simulink model "Experiment_cs"  (Simulink 8.4)
settings: Solver=ode5  SolverMode=SingleTasking  StartTime=0.0  StopTime=inf  FixedStep=1/100  RelTol=1e-3
PreLoadFcn:
  | mbxruntime.callbacks.PreLoadFcn(bdroot);
PostLoadFcn:
  | mbxruntime.callbacks.PostLoadFcn(bdroot);
InitFcn:
  | mbxruntime.callbacks.InitFcn(bdroot);
StartFcn:
  | mbxruntime.callbacks.StartFcn(bdroot);
StopFcn:
  | mbxruntime.callbacks.StopFcn(bdroot);
undefined symbols (not defined in the file or in its folder): dfreq, gray, InitImageOutputDir, Rec, SDTV, strel
libraries: simulink x79, visiontextngfix x30, simulink_extras x23, PreScanSimulinkLibrary x20, visionconversions x6, visionsinks x4, PreScanUsefulBlocks x3, visionstatistics x2, visionmorphops x2, visionanalysis x2, simulink_need_slupdate x2
(part 8 of 11)

== system Experiment_cs/Audi_A8_1/ENABLED/Dynamics_Simple/Chassis/Bicycle_model_[XYZ]/X_Motion ==
  DriveTorque_[Nm] : Inport
  BrakePressure_[bar] : Inport  Port=2
  v0_[ms-1] : Inport  Port=3
  Air&RoadResistance : Subsystem
  BrakeSystem : Subsystem
  Configurable Subsystem : Subsystem  BlockChoice=Integrator  mask{ComputationMode=ComputationMode}
      mask prompts: ComputationMode "Computation mode:"
      mask init:
      | SetComputationMode(gcb,ComputationMode);
      settings: AttributesFormatString=%<BlockChoice>  OpenFcn=BringToFront(gcb);  MemberBlocks=Discrete-Time Integrator,Integrator
      settings: TemplateBlock=|
      | PreScanSimulinkLibrary/Configurable Subsystems/integral with reset and initial condition/Configurable
      | Subsystem
  Configurable Subsystem1 : Subsystem  BlockChoice=Torsional damping  mask{ComputationMode=ComputationMode}
      mask prompts: ComputationMode "Compuation mode:"
      mask init:
      | SetComputationMode(gcb,ComputationMode);
      settings: AttributesFormatString=%<BlockChoice>  OpenFcn=BringToFront(gcb);  MemberBlocks=Discrete Torsional damping,Torsional damping
      settings: TemplateBlock=|
      | PreScanSimulinkLibrary/Configurable Subsystems/TransferFunction
      | Torsional damping/Configurable
      | Subsystem
  Gain : Gain  Gain=1/p.Rw
  Inertia : Gain  Gain=1/p.m  SaturateOnIntegerOverflow=on  OutDataTypeStr=Inherit: Same as input  ParamDataTypeStr=Inherit: Same as input
  Max RPM and zero- velocity detection : Subsystem
  Sum : Sum  Inputs=+-  SaturateOnIntegerOverflow=on  InputSameDT=on  OutDataTypeStr=Inherit: Same as first input
  Sum2 : Sum  Inputs=+-  SaturateOnIntegerOverflow=on  InputSameDT=on  OutDataTypeStr=Inherit: Same as first input
  vx_[ms-1] : Outport
  ax_[ms-2] : Outport  Port=2
  wires:
  Sum/1 -> Sum2/1  "sumForce_[N]"
  Inertia/1 -> Max RPM and zero- velocity detection/1(ax)  "ax[ms-2]"
  Sum2/1 -> Inertia/1
  Air&RoadResistance/1(Resistance_Force) -> Sum/2
  Configurable Subsystem/1(Out1) -> vx_[ms-1]/1, Air&RoadResistance/1(vx_[ms-1]), BrakeSystem/1(vx_[ms-1]), Max RPM and zero- velocity detection/5(vx)  "vx_[ms-1]"
  BrakePressure_[bar]/1 -> BrakeSystem/2(BrakePressure_[bar])  "BrakePressure_[bar]"
  DriveTorque_[Nm]/1 -> Configurable Subsystem1/1(In1)  "DriveTorque_[Nm]"
  Configurable Subsystem1/1(Out1) -> [DT], Gain/1
  Max RPM and zero- velocity detection/1(ax_out) -> Configurable Subsystem/1(In1), ax_[ms-2]/1  "ax [ms-2]"
  Max RPM and zero- velocity detection/2(vx_reset) -> Configurable Subsystem/2(In2)
  Max RPM and zero- velocity detection/3(x0) -> Configurable Subsystem/3(In3)
  v0_[ms-1]/1 -> Max RPM and zero- velocity detection/4(v0)
  [DT] -> Max RPM and zero- velocity detection/2(Drive Torque)
  [BT] -> Max RPM and zero- velocity detection/3(Brake Torque)
  BrakeSystem/1(BrakeForce) -> Sum2/2
  BrakeSystem/2(BrakeTorqueAbs) -> [BT]
  Gain/1 -> Sum/1

== system Experiment_cs/Audi_A8_1/ENABLED/Dynamics_Simple/Chassis/Bicycle_model_[XYZ]/Y & Yaw_Motion ==
  |vx|_[ms-1] : Inport
  Fy_[N] : Inport  Port=2
  Mz_[Nm] : Inport  Port=3
  Compare To Zero : simulink/Logic and Bit Operations/Compare To Zero  relop===  OutDataTypeStr=boolean  ZeroCross=off
  Configurable Subsystem : Subsystem  BlockChoice=Integrator  mask{ComputationMode=ComputationMode}
      mask prompts: ComputationMode "Computation mode:"
      mask init:
      | SetComputationMode(gcb,ComputationMode);
      settings: AttributesFormatString=%<BlockChoice>  OpenFcn=BringToFront(gcb);  MemberBlocks=Discrete-Time Integrator,Integrator
      settings: TemplateBlock=|
      | PreScanSimulinkLibrary/Configurable Subsystems/integral with reset/Configurable
      | Subsystem
  Configurable Subsystem1 : Subsystem  BlockChoice=Integrator  mask{ComputationMode=ComputationMode}
      link override Discrete-Time Integrator: IntegratorMethod=Integration: Backward Euler
      mask prompts: ComputationMode "Computation mode:"
      mask init:
      | SetComputationMode(gcb,ComputationMode);
      settings: AttributesFormatString=%<BlockChoice>  OpenFcn=BringToFront(gcb);  MemberBlocks=Discrete-Time Integrator,Integrator
      settings: TemplateBlock=|
      | PreScanSimulinkLibrary/Configurable Subsystems/integral/Configurable
      | Subsystem1
  Configurable Subsystem2 : Subsystem  BlockChoice=Integrator  mask{ComputationMode=ComputationMode}
      mask prompts: ComputationMode "Computation mode:"
      mask init:
      | SetComputationMode(gcb,ComputationMode);
      settings: AttributesFormatString=%<BlockChoice>  OpenFcn=BringToFront(gcb);  MemberBlocks=Discrete-Time Integrator,Integrator
      settings: TemplateBlock=|
      | PreScanSimulinkLibrary/Configurable Subsystems/integral with reset/Configurable
      | Subsystem
  Fcn1 : Fcn  Expr=u(1)*u(3)
  Gain : Gain  Gain=1/p.m  SaturateOnIntegerOverflow=on  OutDataTypeStr=Inherit: Same as input  ParamDataTypeStr=Inherit: Same as input
  Gain1 : Gain  Gain=1/p.J_zz  SaturateOnIntegerOverflow=on  OutDataTypeStr=Inherit: Same as input  ParamDataTypeStr=Inherit: Same as input
  Sum1 : Sum  Inputs=-+  SaturateOnIntegerOverflow=on  InputSameDT=on  OutDataTypeStr=Inherit: Same as first input
  mux : Mux  Inputs=3
  |vx|_[ms-1]1 : Outport  InitialOutput=0
  vy_[ms-1] : Outport  Port=2  InitialOutput=0
  ay_[ms-2] : Outport  Port=3  InitialOutput=0
  dYawAngle_[rads-1] : Outport  Port=4  InitialOutput=0
  YawAngle_[rad] : Outport  Port=5  InitialOutput=0
  wires:
  Configurable Subsystem2/1(Out1) -> Configurable Subsystem1/1(In1), mux/3, dYawAngle_[rads-1]/1  "dYawAngle_[rads-1]"
  Configurable Subsystem/1(Out1) -> mux/2, vy_[ms-1]/1  "vy_[ms-1]"
  |vx|_[ms-1]/1 -> mux/1, |vx|_[ms-1]1/1, Compare To Zero/1  "|vx|_[ms-1]"
  mux/1 -> Fcn1/1  "|vx|_[ms-1]_vy_[ms-1]_dYawAngle_[rads-1]"
  Fcn1/1 -> Sum1/1  "|vx|*dYawAngle_[ms-2]"
  Sum1/1 -> Configurable Subsystem/1(In1)  "dvy_[ms-2]"
  Fy_[N]/1 -> Gain/1  "Fy_[N]"
  Mz_[Nm]/1 -> Gain1/1  "Mz_[Nm]"
  Configurable Subsystem1/1(Out1) -> YawAngle_[rad]/1
  Compare To Zero/1 -> [reset]
  [reset] -> Configurable Subsystem2/2(In2)
  [reset] -> Configurable Subsystem/2(In2)
  Gain/1 -> ay_[ms-2]/1, Sum1/2  "ddy_[ms-2]"
  Gain1/1 -> Configurable Subsystem2/1(In1)  "ddYawAngle_[rads-2]"

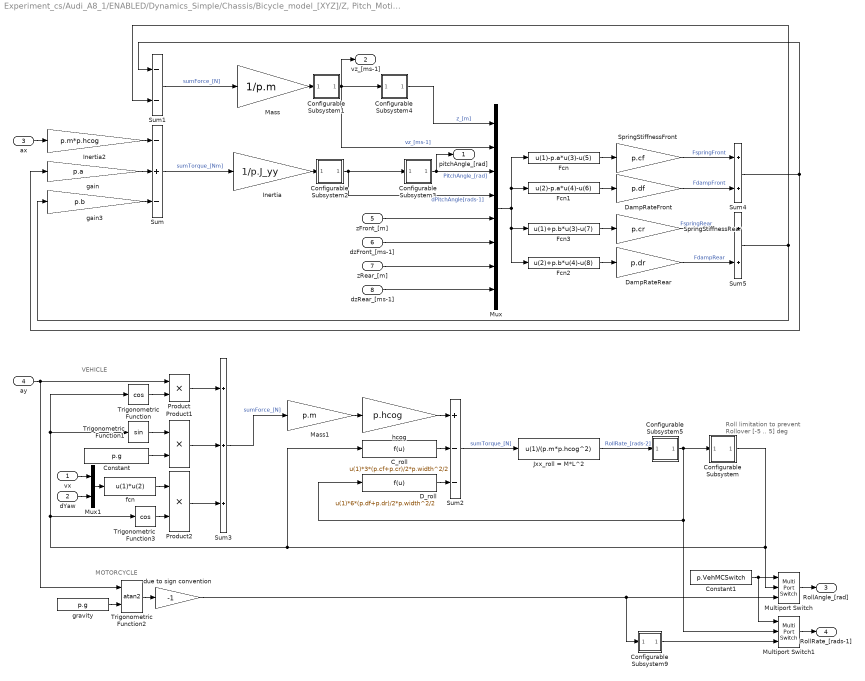
== system Experiment_cs/Audi_A8_1/ENABLED/Dynamics_Simple/Chassis/Bicycle_model_[XYZ]/Z, Pitch_Motion & Roll_Motion ==
  note: MOTORCYCLE
  note: VEHICLE
  note: Roll limitation
      | to prevent
      | Rollover
      | [-5 .. 5] deg
  vx : Inport
  dYaw : Inport  Port=2
  ax : Inport  Port=3
  ay : Inport  Port=4
  zFront_[m] : Inport  Port=5
  dzFront_[ms-1] : Inport  Port=6
  zRear_[m] : Inport  Port=7
  dzRear_[ms-1] : Inport  Port=8
  C_roll : Fcn  Expr=u(1)*3*(p.cf+p.cr)/2*p.width^2/2
  Configurable Subsystem : Subsystem  BlockChoice=Integrator  mask{ComputationMode=ComputationMode}
      link override Discrete-Time Integrator: UpperSaturationLimit=5*pi/180  LowerSaturationLimit=-5*pi/180
      link override Integrator: UpperSaturationLimit=5*pi/180  LowerSaturationLimit=-5*pi/180
      mask prompts: ComputationMode "Computation mode:"
      mask init:
      | SetComputationMode(gcb,ComputationMode);
      settings: AttributesFormatString=%<BlockChoice>  OpenFcn=BringToFront(gcb);  MemberBlocks=Discrete-Time Integrator,Integrator
      settings: TemplateBlock=|
      | PreScanSimulinkLibrary/Configurable Subsystems/integral with limits
      | for roll motion/Configurable
      | Subsystem
  Configurable Subsystem1 : Subsystem  BlockChoice=Integrator  mask{ComputationMode=ComputationMode}
      mask prompts: ComputationMode "Computation mode:"
      mask init:
      | SetComputationMode(gcb,ComputationMode);
      settings: AttributesFormatString=%<BlockChoice>  OpenFcn=BringToFront(gcb);  MemberBlocks=Discrete-Time Integrator,Integrator
      settings: TemplateBlock=|
      | PreScanSimulinkLibrary/Configurable Subsystems/integral/Configurable
      | Subsystem1
  Configurable Subsystem2 : Subsystem  BlockChoice=Integrator  mask{ComputationMode=ComputationMode}
      mask prompts: ComputationMode "Computation mode:"
      mask init:
      | SetComputationMode(gcb,ComputationMode);
      settings: AttributesFormatString=%<BlockChoice>  OpenFcn=BringToFront(gcb);  MemberBlocks=Discrete-Time Integrator,Integrator
      settings: TemplateBlock=|
      | PreScanSimulinkLibrary/Configurable Subsystems/integral/Configurable
      | Subsystem1
  Configurable Subsystem3 : Subsystem  BlockChoice=Integrator  mask{ComputationMode=ComputationMode}
      mask prompts: ComputationMode "Computation mode:"
      mask init:
      | SetComputationMode(gcb,ComputationMode);
      settings: AttributesFormatString=%<BlockChoice>  OpenFcn=BringToFront(gcb);  MemberBlocks=Discrete-Time Integrator,Integrator
      settings: TemplateBlock=|
      | PreScanSimulinkLibrary/Configurable Subsystems/integral/Configurable
      | Subsystem1
  Configurable Subsystem4 : Subsystem  BlockChoice=Integrator  mask{ComputationMode=ComputationMode}
      mask prompts: ComputationMode "Computation mode:"
      mask init:
      | SetComputationMode(gcb,ComputationMode);
      settings: AttributesFormatString=%<BlockChoice>  OpenFcn=BringToFront(gcb);  MemberBlocks=Discrete-Time Integrator,Integrator
      settings: TemplateBlock=|
      | PreScanSimulinkLibrary/Configurable Subsystems/integral/Configurable
      | Subsystem1
  Configurable Subsystem5 : Subsystem  BlockChoice=Integrator  mask{ComputationMode=ComputationMode}
      mask prompts: ComputationMode "Computation mode:"
      mask init:
      | SetComputationMode(gcb,ComputationMode);
      settings: AttributesFormatString=%<BlockChoice>  OpenFcn=BringToFront(gcb);  MemberBlocks=Discrete-Time Integrator,Integrator
      settings: TemplateBlock=|
      | PreScanSimulinkLibrary/Configurable Subsystems/integral/Configurable
      | Subsystem1
  Configurable Subsystem9 : Subsystem  BlockChoice=Derivative  mask{ComputationMode=ComputationMode}
      mask prompts: ComputationMode "Computation mode:"
      mask init:
      | SetComputationMode(gcb,ComputationMode);
      settings: AttributesFormatString=%<BlockChoice>  OpenFcn=BringToFront(gcb);  MemberBlocks=Derivative,Discrete Derivative
      settings: TemplateBlock=|
      | PreScanSimulinkLibrary/Configurable Subsystems/Derivative/Configurable
      | Subsystem
  Constant : Constant  Value=p.g
  Constant1 : Constant  Value=p.VehMCSwitch
  D_roll : Fcn  Expr=u(1)*6*(p.df+p.dr)/2*p.width^2/2
  DampRateFront : Gain  Gain=p.df  SaturateOnIntegerOverflow=on  OutDataTypeStr=Inherit: Same as input  ParamDataTypeStr=Inherit: Same as input
  DampRateRear : Gain  Gain=p.dr  SaturateOnIntegerOverflow=on  OutDataTypeStr=Inherit: Same as input  ParamDataTypeStr=Inherit: Same as input
  Fcn : Fcn  Expr=u(1)-p.a*u(3)-u(5)
  Fcn1 : Fcn  Expr=u(2)-p.a*u(4)-u(6)
  Fcn2 : Fcn  Expr=u(2)+p.b*u(4)-u(8)
  Fcn3 : Fcn  Expr=u(1)+p.b*u(3)-u(7)
  Inertia : Gain  Gain=1/p.J_yy  SaturateOnIntegerOverflow=on  OutDataTypeStr=Inherit: Same as input  ParamDataTypeStr=Inherit: Same as input
  Inertia2 : Gain  Gain=p.m*p.hcog  SaturateOnIntegerOverflow=on  OutDataTypeStr=Inherit: Same as input  ParamDataTypeStr=Inherit: Same as input
  Jxx_roll = M*L^2 : Fcn  Expr=u(1)/(p.m*p.hcog^2)
  Mass : Gain  Gain=1/p.m  SaturateOnIntegerOverflow=on  OutDataTypeStr=Inherit: Same as input  ParamDataTypeStr=Inherit: Same as input
  Mass1 : Gain  Gain=p.m  SaturateOnIntegerOverflow=on  OutDataTypeStr=Inherit: Same as input  ParamDataTypeStr=Inherit: Same as input
  Multiport Switch : MultiPortSwitch  Inputs=2
  Multiport Switch1 : MultiPortSwitch  Inputs=2
  Mux : Mux  Inputs=8
  Mux1 : Mux  Inputs=2
  Product : Product  RndMeth=Zero
  Product1 : Product  RndMeth=Zero
  Product2 : Product  RndMeth=Zero
  SpringStiffnessFront : Gain  Gain=p.cf  SaturateOnIntegerOverflow=on  OutDataTypeStr=Inherit: Same as input  ParamDataTypeStr=Inherit: Same as input
  SpringStiffnessRear : Gain  Gain=p.cr  SaturateOnIntegerOverflow=on  OutDataTypeStr=Inherit: Same as input  ParamDataTypeStr=Inherit: Same as input
  Sum : Sum  Inputs=-+-  SaturateOnIntegerOverflow=on  InputSameDT=on  OutDataTypeStr=Inherit: Same as first input
  Sum1 : Sum  Inputs=--  SaturateOnIntegerOverflow=on  InputSameDT=on  OutDataTypeStr=Inherit: Same as first input
  Sum2 : Sum  Inputs=+--  SaturateOnIntegerOverflow=on  InputSameDT=on  OutDataTypeStr=Inherit: Same as first input
  Sum3 : Sum  Inputs=+++  SaturateOnIntegerOverflow=on  InputSameDT=on  OutDataTypeStr=Inherit: Same as first input
  Sum4 : Sum  SaturateOnIntegerOverflow=on  InputSameDT=on  OutDataTypeStr=Inherit: Same as first input
  Sum5 : Sum  SaturateOnIntegerOverflow=on  InputSameDT=on  OutDataTypeStr=Inherit: Same as first input
  Trigonometric Function : Trigonometry  Operator=cos
  Trigonometric Function1 : Trigonometry
  Trigonometric Function2 : Trigonometry  Operator=atan2
  Trigonometric Function3 : Trigonometry  Operator=cos
  due to sign convention : Gain  Gain=-1  SaturateOnIntegerOverflow=on  OutDataTypeStr=Inherit: Same as input  ParamDataTypeStr=Inherit: Same as input
  fcn : Fcn  Expr=u(1)*u(2)
  gain : Gain  Gain=p.a  SaturateOnIntegerOverflow=on  OutDataTypeStr=Inherit: Same as input  ParamDataTypeStr=Inherit: Same as input
  gain3 : Gain  Gain=p.b  SaturateOnIntegerOverflow=on  OutDataTypeStr=Inherit: Same as input  ParamDataTypeStr=Inherit: Same as input
  gravity : Constant  Value=p.g
  hcog : Gain  Gain=p.hcog  SaturateOnIntegerOverflow=on  OutDataTypeStr=Inherit: Same as input  ParamDataTypeStr=Inherit: Same as input
  pitchAngle_[rad] : Outport
  vz_[ms-1] : Outport  Port=2
  RollAngle_[rad] : Outport  Port=3
  RollRate_[rads-1] : Outport  Port=4
  wires:
  Inertia/1 -> Configurable Subsystem2/1(In1)
  Configurable Subsystem2/1(Out1) -> Configurable Subsystem3/1(In1), Mux/4  "dPitchAngle[rads-1]"
  Mass/1 -> Configurable Subsystem1/1(In1)
  Configurable Subsystem1/1(Out1) -> Configurable Subsystem4/1(In1), Mux/2, vz_[ms-1]/1  "vz_[ms-1]"
  ax/1 -> Inertia2/1
  Inertia2/1 -> Sum/1
  zFront_[m]/1 -> Mux/5
  dzFront_[ms-1]/1 -> Mux/6
  zRear_[m]/1 -> Mux/7
  dzRear_[ms-1]/1 -> Mux/8
  Configurable Subsystem4/1(Out1) -> Mux/1  "z_[m]"
  SpringStiffnessFront/1 -> Sum4/1  "FspringFront"
  DampRateFront/1 -> Sum4/2  "FdampFront"
  DampRateRear/1 -> Sum5/2  "FdampRear"
  SpringStiffnessRear/1 -> Sum5/1  "FspringRear"
  gain3/1 -> Sum/3
  gain/1 -> Sum/2
  Configurable Subsystem3/1(Out1) -> Mux/3, pitchAngle_[rad]/1  "PitchAngle_[rad]"
  Sum4/1 -> Sum1/1, gain/1
  Sum5/1 -> gain3/1, Sum1/2
  Sum2/1 -> Jxx_roll = M*L^2/1  "sumTorque_[N]"
  Jxx_roll = M*L^2/1 -> Configurable Subsystem5/1(In1)  "RollRate_[rads-2]"
  Configurable Subsystem5/1(Out1) -> Configurable Subsystem/1(In1), D_roll/1, Multiport Switch1/2
  Configurable Subsystem/1(Out1) -> C_roll/1, Trigonometric Function1/1, Trigonometric Function/1, Trigonometric Function3/1, Multiport Switch/2
  Trigonometric Function/1 -> Product/2
  ay/1 -> Product/1, Trigonometric Function2/1
  Trigonometric Function1/1 -> Product1/1
  Constant/1 -> Product1/2
  Product/1 -> Sum3/1
  Product1/1 -> Sum3/2
  Mass1/1 -> hcog/1
  hcog/1 -> Sum2/1
  C_roll/1 -> Sum2/2
  D_roll/1 -> Sum2/3
  Mux/1 -> Fcn2/1, Fcn3/1, Fcn/1, Fcn1/1
  Fcn/1 -> SpringStiffnessFront/1
  Fcn1/1 -> DampRateFront/1
  Fcn3/1 -> SpringStiffnessRear/1
  Fcn2/1 -> DampRateRear/1
  due to sign convention/1 -> Configurable Subsystem9/1(In1), Multiport Switch/3
  Trigonometric Function2/1 -> due to sign convention/1
  gravity/1 -> Trigonometric Function2/2
  Constant1/1 -> Multiport Switch/1, Multiport Switch1/1
  Multiport Switch/1 -> RollAngle_[rad]/1
  Multiport Switch1/1 -> RollRate_[rads-1]/1
  Configurable Subsystem9/1(Out1) -> Multiport Switch1/3
  Mux1/1 -> fcn/1
  vx/1 -> Mux1/1
  dYaw/1 -> Mux1/2
  fcn/1 -> Product2/1
  Trigonometric Function3/1 -> Product2/2
  Product2/1 -> Sum3/3
  Sum/1 -> Inertia/1  "sumTorque_[Nm]"
  Sum1/1 -> Mass/1  "sumForce_[N]"
  Sum3/1 -> Mass1/1  "sumForce_[N]"

== system Experiment_cs/Audi_A8_1/ENABLED/Dynamics_Simple/Chassis/FrontTyre/AlphaFront ==
  In : Inport
  Abs : Abs
  Compare To Constant : simulink/Logic and Bit Operations/Compare To Constant  relop=>  const=0  OutDataTypeStr=uint8  ZeroCross=off
  Enabled Subsystem : Subsystem  TreatAsAtomicUnit=on
  Selector : Selector
  Alpha : Outport
  wires:
  Selector/1 -> Abs/1
  Compare To Constant/1 -> Enabled Subsystem/Enable
  Enabled Subsystem/1(Alpha) -> Alpha/1
  In/1 -> Enabled Subsystem/1(In), Selector/1
  Abs/1 -> Compare To Constant/1

== system Experiment_cs/Audi_A8_1/ENABLED/Dynamics_Simple/Chassis/FrontTyre/Configurable Subsystem ==
  In1 : Inport
  In2 : Inport  Port=2
  Integrator : Integrator  ExternalReset=level  LimitOutput=on  UpperSaturationLimit=1  LowerSaturationLimit=-1
  Out1 : Outport
  wires:
  In1/1 -> Integrator/1
  In2/1 -> Integrator/2
  Integrator/1 -> Out1/1

== system Experiment_cs/Audi_A8_1/ENABLED/Dynamics_Simple/Chassis/FrontTyre/Configurable Subsystem1 ==
  In1 : Inport
  In2 : Inport  Port=2
  Integrator : Integrator  ExternalReset=level
  Out1 : Outport
  wires:
  In1/1 -> Integrator/1
  In2/1 -> Integrator/2
  Integrator/1 -> Out1/1

== system Experiment_cs/Audi_A8_1/ENABLED/Dynamics_Simple/Chassis/FrontTyre/Prevent_instability_at_low_Vx ==
  note: |vx|
  alpha[rad] : Inport
  In : Inport  Port=2
  Divide : Product  Inputs=**
  Lookup Table : Lookup  InputValues="[0    2.5   ]"  Table="[0.01    1]"  LookUpMeth=Interpolation-Use End Values
  Selector : Selector  InputPortWidth=3  Indices=[1]
  alpha [rad] : Outport
  wires:
  In/1 -> Selector/1
  Lookup Table/1 -> Divide/2
  Selector/1 -> Lookup Table/1
  alpha[rad]/1 -> Divide/1
  Divide/1 -> alpha [rad]/1

== system Experiment_cs/Audi_A8_1/ENABLED/Dynamics_Simple/Chassis/MuxDynState/Configurable Subsystem1 ==
  In1 : Inport
  Integrator : Integrator
  Out1 : Outport
  wires:
  In1/1 -> Integrator/1
  Integrator/1 -> Out1/1

== system Experiment_cs/Audi_A8_1/ENABLED/Dynamics_Simple/Chassis/MuxDynState/Transformation_BODY2GLOBAL ==
  Vvector_BODY_[m/s] : Inport
  angles_BODYwrtGLOB_[rad] : Inport  Port=2
  Dot Product : DotProduct  InputSameDT=on  OutDataTypeStr=Inherit: Inherit via internal rule
  Dot Product1 : DotProduct  InputSameDT=on  OutDataTypeStr=Inherit: Inherit via internal rule
  Dot Product2 : DotProduct  InputSameDT=on  OutDataTypeStr=Inherit: Inherit via internal rule
  Fcn10 : Fcn  Expr=cos(u(1))*sin(u(2))*sin(u(3))-sin(u(1))*cos(u(3))
  Fcn11 : Fcn  Expr=cos(u(1))*sin(u(2))*cos(u(3))+sin(u(1))*sin(u(3))
  Fcn12 : Fcn  Expr=sin(u(1))*cos(u(2))
  Fcn13 : Fcn  Expr=sin(u(1))*sin(u(2))*sin(u(3))+cos(u(1))*cos(u(3))
  Fcn14 : Fcn  Expr=sin(u(1))*sin(u(2))*cos(u(3))-cos(u(1))*sin(u(3))
  Fcn15 : Fcn  Expr=-sin(u(2))
  Fcn16 : Fcn  Expr=cos(u(2))*sin(u(3))
  Fcn17 : Fcn  Expr=cos(u(2))*cos(u(3))
  Fcn9 : Fcn  Expr=cos(u(1))*cos(u(2))
  Mux1 : Mux  Inputs=9
  Mux3 : Mux  Inputs=3
  Selector : Selector  InputPortWidth=9  Indices=[1 2 3]
  Selector1 : Selector  InputPortWidth=9  Indices=[4 5 6]
  Selector2 : Selector  InputPortWidth=9  Indices=[7 8 9]
  rot_xyz 2 rot_zyx : Selector  InputPortWidth=3  Indices=[3 2 1]
  Vvector_GLOBAL_[m/s] : Outport
  wires:
  Fcn9/1 -> Mux1/1
  Fcn10/1 -> Mux1/2
  Fcn11/1 -> Mux1/3
  Fcn12/1 -> Mux1/4
  Fcn13/1 -> Mux1/5
  Fcn14/1 -> Mux1/6
  Fcn15/1 -> Mux1/7
  Fcn16/1 -> Mux1/8
  Fcn17/1 -> Mux1/9
  Mux1/1 -> Selector/1, Selector1/1, Selector2/1  "RotationMatrix Visu"
  Selector/1 -> Dot Product/2
  Vvector_BODY_[m/s]/1 -> Dot Product2/1, Dot Product1/1, Dot Product/1
  Dot Product/1 -> Mux3/1
  Selector1/1 -> Dot Product1/2
  Selector2/1 -> Dot Product2/2
  Dot Product2/1 -> Mux3/3
  Dot Product1/1 -> Mux3/2
  rot_xyz 2 rot_zyx/1 -> Fcn9/1, Fcn10/1, Fcn11/1, Fcn12/1, Fcn13/1, Fcn14/1, Fcn15/1, Fcn16/1, Fcn17/1
  Mux3/1 -> Vvector_GLOBAL_[m/s]/1
  angles_BODYwrtGLOB_[rad]/1 -> rot_xyz 2 rot_zyx/1

== system Experiment_cs/Audi_A8_1/ENABLED/Dynamics_Simple/Chassis/RearTyre/AlphaRear ==
  In : Inport
  Abs : Abs
  Compare To Constant : simulink/Logic and Bit Operations/Compare To Constant  relop=>  const=0  OutDataTypeStr=uint8  ZeroCross=off
  Enabled Subsystem : Subsystem  TreatAsAtomicUnit=on
  Selector : Selector
  Alpha : Outport
  wires:
  Selector/1 -> Abs/1
  Compare To Constant/1 -> Enabled Subsystem/Enable
  Enabled Subsystem/1(Alpha) -> Alpha/1
  In/1 -> Enabled Subsystem/1(In), Selector/1
  Abs/1 -> Compare To Constant/1

== system Experiment_cs/Audi_A8_1/ENABLED/Dynamics_Simple/Chassis/RearTyre/Configurable Subsystem ==
  In1 : Inport
  In2 : Inport  Port=2
  Integrator : Integrator  ExternalReset=level
  Out1 : Outport
  wires:
  In1/1 -> Integrator/1
  In2/1 -> Integrator/2
  Integrator/1 -> Out1/1

== system Experiment_cs/Audi_A8_1/ENABLED/Dynamics_Simple/Chassis/RearTyre/Configurable Subsystem1 ==
  In1 : Inport
  In2 : Inport  Port=2
  Integrator : Integrator  ExternalReset=level  LimitOutput=on  UpperSaturationLimit=1  LowerSaturationLimit=-1
  Out1 : Outport
  wires:
  In1/1 -> Integrator/1
  In2/1 -> Integrator/2
  Integrator/1 -> Out1/1

== system Experiment_cs/Audi_A8_1/ENABLED/Dynamics_Simple/ShiftLogic/Detect Increase/If V0 higher of the from 2->3 shifting velocity ==
  In1 : Inport
  Action Port : ActionPort  PropagateVarSize=During execution  ActionType=then
  Out1 : Outport
  wires:
  In1/1 -> Out1/1

== system Experiment_cs/Audi_A8_1/ENABLED/Dynamics_Simple/ShiftLogic/Detect Increase/Other ==
  In1 : Inport
  Action Port : ActionPort  PropagateVarSize=During execution  ActionType=else
  Data Type Conversion : DataTypeConversion  OutDataTypeStr=double
  Detect Increase : simulink/Logic and Bit Operations/Detect Increase  vinit=0.0  InputProcessing=Inherited  OutDataTypeStr=uint8
  Out1 : Outport
  wires:
  In1/1 -> Detect Increase/1
  Detect Increase/1 -> Data Type Conversion/1
  Data Type Conversion/1 -> Out1/1

== system Experiment_cs/Audi_A8_1/ENABLED/Dynamics_Simple/Transmission/Transmission_Ratio/If Action Neutral ==
  In1 : Inport
  Action Port : ActionPort  InitializeStates=reset  PropagateVarSize=During execution  ActionType=then
  Out1 : Outport
  wires:
  In1/1 -> Out1/1

== system Experiment_cs/Audi_A8_1/ENABLED/Dynamics_Simple/Transmission/Transmission_Ratio/If Action Normal ==
  In1 : Inport
  Action Port : ActionPort  InitializeStates=reset  PropagateVarSize=During execution  ActionType=else
  Out1 : Outport
  wires:
  In1/1 -> Out1/1

== system Experiment_cs/Audi_A8_1/ENABLED/Dynamics_Simple/Transmission/Transmission_Ratio/If Action Reverse ==
  In1 : Inport
  Action Port : ActionPort  InitializeStates=reset  PropagateVarSize=During execution  ActionType=elseif
  Reverse : Gain  Gain=-1
  Out1 : Outport
  wires:
  Reverse/1 -> Out1/1
  In1/1 -> Reverse/1

== system Experiment_cs/Audi_A8_1/ENABLED/PPS Model/Pedestrian detection/Blob Analysis/Transpose ==
  U : Inport
  Data Type Conversion : DataTypeConversion
  Data Type Conversion1 : DataTypeConversion  OutDataTypeStr=single
  Interpreted MATLAB Function : MATLABFcn  MATLABFcn=transpose  Output1D=off
  Y : Outport
  wires:
  Data Type Conversion1/1 -> Y/1
  Interpreted MATLAB Function/1 -> Data Type Conversion1/1
  Data Type Conversion/1 -> Interpreted MATLAB Function/1
  U/1 -> Data Type Conversion/1

== system Experiment_cs/Audi_A8_1/ENABLED/PPS Model/Pedestrian detection/Blob Analysis/Transpose1 ==
  U : Inport
  Data Type Conversion : DataTypeConversion
  Data Type Conversion1 : DataTypeConversion  OutDataTypeStr=int32
  Interpreted MATLAB Function : MATLABFcn  MATLABFcn=transpose  Output1D=off
  Y : Outport
  wires:
  U/1 -> Data Type Conversion/1
  Data Type Conversion/1 -> Interpreted MATLAB Function/1
  Interpreted MATLAB Function/1 -> Data Type Conversion1/1
  Data Type Conversion1/1 -> Y/1

== system Experiment_cs/Audi_A8_1/ENABLED/PPS Model/Pedestrian detection/Blob Analysis/Transpose2 ==
  U : Inport
  Data Type Conversion : DataTypeConversion
  Data Type Conversion1 : DataTypeConversion  OutDataTypeStr=single
  Interpreted MATLAB Function : MATLABFcn  MATLABFcn=transpose  Output1D=off
  Y : Outport
  wires:
  U/1 -> Data Type Conversion/1
  Data Type Conversion/1 -> Interpreted MATLAB Function/1
  Interpreted MATLAB Function/1 -> Data Type Conversion1/1
  Data Type Conversion1/1 -> Y/1

== system Experiment_cs/Audi_A8_1/ENABLED/PPS Model/Pedestrian detection/Blob Analysis/Transpose3 ==
  U : Inport
  Data Type Conversion : DataTypeConversion
  Data Type Conversion1 : DataTypeConversion
  Interpreted MATLAB Function : MATLABFcn  MATLABFcn=transpose  Output1D=off
  Y : Outport
  wires:
  Data Type Conversion1/1 -> Y/1
  Interpreted MATLAB Function/1 -> Data Type Conversion1/1
  Data Type Conversion/1 -> Interpreted MATLAB Function/1
  U/1 -> Data Type Conversion/1

== system Experiment_cs/Audi_A8_1/ENABLED/PPS Model/Pedestrian detection/Blob Analysis/Transpose4 ==
  U : Inport
  Data Type Conversion : DataTypeConversion
  Data Type Conversion1 : DataTypeConversion  OutDataTypeStr=int32
  Interpreted MATLAB Function : MATLABFcn  MATLABFcn=transpose  Output1D=off
  Y : Outport
  wires:
  U/1 -> Data Type Conversion/1
  Data Type Conversion/1 -> Interpreted MATLAB Function/1
  Interpreted MATLAB Function/1 -> Data Type Conversion1/1
  Data Type Conversion1/1 -> Y/1

== system Experiment_cs/Audi_A8_1/ENABLED/PPS Model/Pedestrian detection/Blob Analysis/Transpose5 ==
  U : Inport
  Data Type Conversion : DataTypeConversion
  Data Type Conversion1 : DataTypeConversion  OutDataTypeStr=single
  Interpreted MATLAB Function : MATLABFcn  MATLABFcn=transpose  Output1D=off
  Y : Outport
  wires:
  Data Type Conversion1/1 -> Y/1
  Interpreted MATLAB Function/1 -> Data Type Conversion1/1
  Data Type Conversion/1 -> Interpreted MATLAB Function/1
  U/1 -> Data Type Conversion/1

== system Experiment_cs/Audi_A8_1/ENABLED/PPS Model/Pedestrian detection/Blob Analysis/Transpose6 ==
  U : Inport
  Data Type Conversion : DataTypeConversion
  Data Type Conversion1 : DataTypeConversion  OutDataTypeStr=single
  Interpreted MATLAB Function : MATLABFcn  MATLABFcn=transpose  Output1D=off
  Y : Outport
  wires:
  U/1 -> Data Type Conversion/1
  Data Type Conversion/1 -> Interpreted MATLAB Function/1
  Interpreted MATLAB Function/1 -> Data Type Conversion1/1
  Data Type Conversion1/1 -> Y/1

== system Experiment_cs/Audi_A8_1/ENABLED/PPS Model/Pedestrian detection/Blob Analysis/Transpose7 ==
  U : Inport
  Data Type Conversion : DataTypeConversion
  Data Type Conversion1 : DataTypeConversion  OutDataTypeStr=single
  Interpreted MATLAB Function : MATLABFcn  MATLABFcn=transpose  Output1D=off
  Y : Outport
  wires:
  U/1 -> Data Type Conversion/1
  Data Type Conversion/1 -> Interpreted MATLAB Function/1
  Interpreted MATLAB Function/1 -> Data Type Conversion1/1
  Data Type Conversion1/1 -> Y/1

== system Experiment_cs/Audi_A8_1/ENABLED/PPS Model/Radar detection/Bend road segment/Lead Car Longitudinal Velocity1 ==
  TIS Rangedot [m/s] : Inport
  theta [rad] : Inport  Port=2
  lambda [rad] : Inport  Port=3
  Add1 : Sum  Inputs=+-
  Constant : Constant  Value=0
  Divide2 : Product  Inputs=*/
  Switch1 : Switch  Criteria=u2 ~= 0
  TIS1 Rangedot [m/s]1 : InportShadow
  Trigonometric Function : Trigonometry  Operator=cos
  Vw [m/s] : Outport
  wires:
  TIS Rangedot [m/s]/1 -> Divide2/1
  lambda [rad]/1 -> Add1/1
  theta [rad]/1 -> Add1/2
  Add1/1 -> Trigonometric Function/1
  Trigonometric Function/1 -> Divide2/2
  Divide2/1 -> Switch1/1
  Switch1/1 -> Vw [m/s]/1
  TIS1 Rangedot [m/s]1/1 -> Switch1/2
  Constant/1 -> Switch1/3

== system Experiment_cs/Audi_A8_1/ENABLED/PPS Model/Radar detection/Bend road segment/Saturation1 ==
  TTCin : Inport
  TTCdem_in : Inport  Port=2  SampleTime=1/TISfreq
  Compare To Zero : simulink/Logic and Bit Operations/Compare To Zero  relop=<=  OutDataTypeStr=uint8
  Gain : Gain  Gain=2
  Gain1 : Gain  Gain=ones(TISdet,1)
  Logical Operator : Logic  Operator=OR  AllPortsSameDT=off  OutDataTypeStr=boolean
  Relational Operator : RelationalOperator  Operator=>  OutDataTypeStr=boolean
  Switch : Switch  Criteria=u2 > Threshold  Threshold=0.5
  TTCout : Outport
  TTCdem_out : Outport  Port=2
  wires:
  Gain/1 -> Switch/1, Relational Operator/2
  Gain1/1 -> Gain/1, TTCdem_out/1
  Switch/1 -> TTCout/1
  TTCdem_in/1 -> Gain1/1
  Compare To Zero/1 -> Logical Operator/1
  Relational Operator/1 -> Logical Operator/2
  Logical Operator/1 -> Switch/2
  TTCin/1 -> Switch/3, Compare To Zero/1, Relational Operator/1

== system Experiment_cs/Audi_A8_1/ENABLED/PPS Model/Radar detection/Bend road segment/Saturation2 ==
  TTCin : Inport
  TTCdem_in : Inport  Port=2  SampleTime=1/TISfreq
  Compare To Zero : simulink/Logic and Bit Operations/Compare To Zero  relop=<=  OutDataTypeStr=uint8
  Gain : Gain  Gain=2
  Gain1 : Gain  Gain=ones(TISdet,1)
  Logical Operator : Logic  Operator=OR  AllPortsSameDT=off  OutDataTypeStr=boolean
  Relational Operator : RelationalOperator  Operator=>  OutDataTypeStr=boolean
  Switch : Switch  Criteria=u2 > Threshold  Threshold=0.5
  TTCout : Outport
  TTCdem_out : Outport  Port=2
  wires:
  TTCin/1 -> Relational Operator/1, Compare To Zero/1, Switch/3
  Logical Operator/1 -> Switch/2
  Relational Operator/1 -> Logical Operator/2
  Compare To Zero/1 -> Logical Operator/1
  TTCdem_in/1 -> Gain1/1
  Switch/1 -> TTCout/1
  Gain1/1 -> TTCdem_out/1, Gain/1
  Gain/1 -> Relational Operator/2, Switch/1

== system Experiment_cs/Audi_A8_1/ENABLED/PPS Model/Radar detection/Bend road segment/Saturation3 ==
  TTCin : Inport
  TTCdem_in : Inport  Port=2  SampleTime=1/TISfreq
  Compare To Zero : simulink/Logic and Bit Operations/Compare To Zero  relop=<=  OutDataTypeStr=uint8
  Gain : Gain  Gain=2
  Gain1 : Gain  Gain=ones(TISdet,1)
  Logical Operator : Logic  Operator=OR  AllPortsSameDT=off  OutDataTypeStr=boolean
  Relational Operator : RelationalOperator  Operator=>  OutDataTypeStr=boolean
  Switch : Switch  Criteria=u2 > Threshold  Threshold=0.5
  TTCout : Outport
  TTCdem_out : Outport  Port=2
  wires:
  TTCin/1 -> Relational Operator/1, Compare To Zero/1, Switch/3
  Logical Operator/1 -> Switch/2
  Relational Operator/1 -> Logical Operator/2
  Compare To Zero/1 -> Logical Operator/1
  TTCdem_in/1 -> Gain1/1
  Switch/1 -> TTCout/1
  Gain1/1 -> TTCdem_out/1, Gain/1
  Gain/1 -> Relational Operator/2, Switch/1

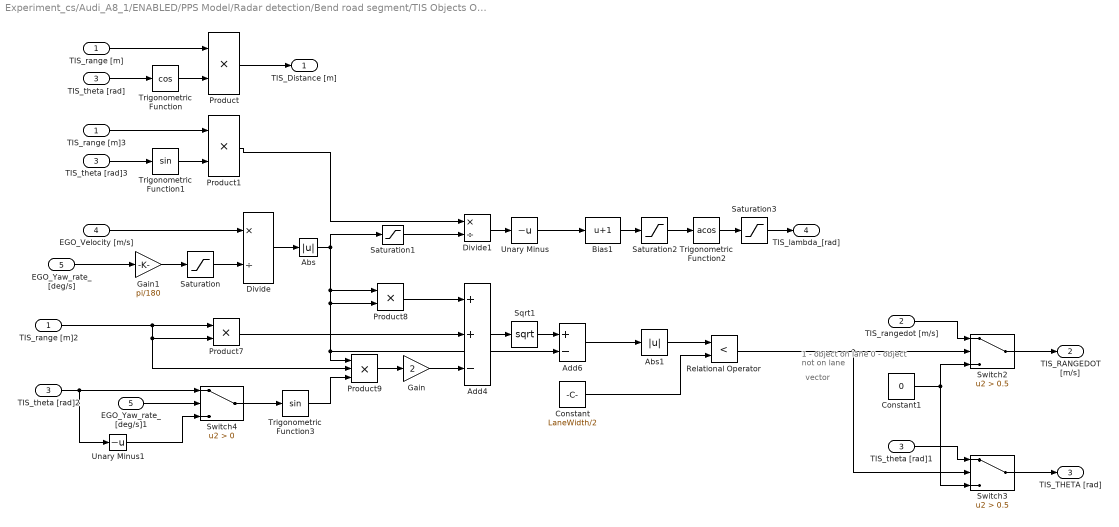
== system Experiment_cs/Audi_A8_1/ENABLED/PPS Model/Radar detection/Bend road segment/TIS Objects On Bend Road ==
  note: 1  - object      on lane
      | 0 - object not on lane
  note: vector
  TIS_range [m] : Inport
  TIS_rangedot [m/s] : Inport  Port=2
  TIS_theta [rad] : Inport  Port=3
  EGO_Velocity [m/s] : Inport  Port=4
  EGO_Yaw_rate_[deg/s] : Inport  Port=5
  Abs : Abs
  Abs1 : Abs
  Add4 : Sum  Inputs=++-
  Add6 : Sum  Inputs=+-
  Bias1 : Bias  Bias=1
  Constant : Constant  Value=LaneWidth/2
  Constant1 : Constant  Value=0
  Divide : Product  Inputs=*/
  Divide1 : Product  Inputs=*/
  EGO_Yaw_rate_[deg/s]1 : InportShadow  Port=5
  Gain : Gain  Gain=2
  Gain1 : Gain  Gain=pi/180
  Product{,1,7..8} (4 alike) : Product  RndMeth=Zero
  Product9 : Product  Inputs=3  RndMeth=Zero
  Relational Operator : RelationalOperator  Operator=<  OutDataTypeStr=boolean
  Saturation : Saturate  UpperLimit=inf  LowerLimit=1e-6
  Saturation1 : Saturate  UpperLimit=inf  LowerLimit=1e-6
  Saturation2 : Saturate  UpperLimit=1  LowerLimit=-1
  Saturation3 : Saturate  UpperLimit=pi  LowerLimit=0
  Sqrt1 : Math  Operator=sqrt  SaturateOnIntegerOverflow=on
  Switch2 : Switch  Criteria=u2 > Threshold  Threshold=0.5
  Switch3 : Switch  Criteria=u2 > Threshold  Threshold=0.5
  Switch4 : Switch  Criteria=u2 > Threshold
  TIS_range [m]2 : InportShadow
  TIS_range [m]3 : InportShadow
  TIS_theta [rad]1 : InportShadow  Port=3
  TIS_theta [rad]2 : InportShadow  Port=3
  TIS_theta [rad]3 : InportShadow  Port=3
  Trigonometric Function : Trigonometry  Operator=cos
  Trigonometric Function1 : Trigonometry
  Trigonometric Function2 : Trigonometry  Operator=acos
  Trigonometric Function3 : Trigonometry
  Unary Minus : UnaryMinus
  Unary Minus1 : UnaryMinus
  TIS_Distance [m] : Outport
  TIS_RANGEDOT [m/s] : Outport  Port=2
  TIS_THETA [rad] : Outport  Port=3
  TIS_lambda_[rad] : Outport  Port=4
  wires:
  TIS_range [m]/1 -> Product/1
  TIS_theta [rad]/1 -> Trigonometric Function/1
  Trigonometric Function/1 -> Product/2
  Trigonometric Function1/1 -> Product1/2
  EGO_Velocity [m/s]/1 -> Divide/1
  EGO_Yaw_rate_[deg/s]/1 -> Gain1/1
  Divide/1 -> Abs/1
  Relational Operator/1 -> Switch2/2, Switch3/2
  TIS_rangedot [m/s]/1 -> Switch2/1
  TIS_theta [rad]1/1 -> Switch3/1
  Constant1/1 -> Switch2/3, Switch3/3
  Switch2/1 -> TIS_RANGEDOT [m/s]/1
  Switch3/1 -> TIS_THETA [rad]/1
  Bias1/1 -> Saturation2/1
  Divide1/1 -> Unary Minus/1
  Unary Minus/1 -> Bias1/1
  Trigonometric Function2/1 -> Saturation3/1
  Abs/1 -> Product8/1, Product8/2, Product9/1, Add6/2, Saturation1/1
  Product/1 -> TIS_Distance [m]/1
  Product8/1 -> Add4/1
  Product7/1 -> Add4/2
  Gain/1 -> Add4/3
  Product9/1 -> Gain/1
  Trigonometric Function3/1 -> Product9/3
  Add4/1 -> Sqrt1/1
  Sqrt1/1 -> Add6/1
  Add6/1 -> Abs1/1
  EGO_Yaw_rate_[deg/s]1/1 -> Switch4/2
  Switch4/1 -> Trigonometric Function3/1
  TIS_theta [rad]2/1 -> Unary Minus1/1, Switch4/1
  TIS_range [m]2/1 -> Product7/1, Product7/2, Product9/2
  TIS_range [m]3/1 -> Product1/1
  TIS_theta [rad]3/1 -> Trigonometric Function1/1
  Product1/1 -> Divide1/1
  Abs1/1 -> Relational Operator/1
  Constant/1 -> Relational Operator/2
  Saturation/1 -> Divide/2
  Saturation1/1 -> Divide1/2
  Saturation2/1 -> Trigonometric Function2/1
  Saturation3/1 -> TIS_lambda_[rad]/1
  Gain1/1 -> Saturation/1
  Unary Minus1/1 -> Switch4/3

== system Experiment_cs/Audi_A8_1/ENABLED/PPS Model/Radar detection/Bend road segment/TTC Computing1 ==
  Distance [m] : Inport
  Velocity [m/s] : Inport  Port=2
  Compare : simulink/Logic and Bit Operations/Compare To Constant  relop===  const=1e-6  OutDataTypeStr=uint8  ZeroCross=off
  Constant : Constant  Value=0
  Data Type Conversion : DataTypeConversion  OutDataTypeStr=double
  Product : Product  Inputs=*/  RndMeth=Zero
  Saturation : Saturate  UpperLimit=inf  LowerLimit=1e-6
  Switch : Switch  Criteria=u2 > Threshold
  Switch1 : Switch  Criteria=u2 > Threshold  Threshold=0.5
  TTC [s] : Outport
  wires:
  Velocity [m/s]/1 -> Switch/2, Switch/1
  Constant/1 -> Switch/3, Switch1/1
  Switch/1 -> Saturation/1
  Distance [m]/1 -> Product/1
  Saturation/1 -> Product/2, Compare/1
  Compare/1 -> Data Type Conversion/1
  Product/1 -> Switch1/3
  Switch1/1 -> TTC [s]/1
  Data Type Conversion/1 -> Switch1/2

== system Experiment_cs/Audi_A8_1/ENABLED/PPS Model/Radar detection/Straight road segment/Impact point2 ==
  alfa : Inport
  xp [m] : Inport  Port=2
  yp [m] : Inport  Port=3
  Abs : Abs
  Add : Sum  Inputs=+-
  Compare To Constant : simulink/Logic and Bit Operations/Compare To Constant  relop=<  const=-1e-6  OutDataTypeStr=uint8  ZeroCross=off
  Compare To Constant1 : simulink/Logic and Bit Operations/Compare To Constant  relop=>  const=1e-6  OutDataTypeStr=uint8  ZeroCross=off
  Constant : Constant  Value=0
  Divide : Product  Inputs=*/
  Logical Operator : Logic  Operator=OR  AllPortsSameDT=off  OutDataTypeStr=boolean
  Saturation : Saturate  UpperLimit=inf  LowerLimit=1e-6
  Saturation1 : Saturate  UpperLimit=-1e-6  LowerLimit=-inf
  Saturation2 : Saturate  UpperLimit=300  LowerLimit=0
  Switch : Switch  Criteria=u2 > Threshold  Threshold=LaneWidth/2
  Switch1 : Switch  Criteria=u2 > Threshold  Threshold=0.5
  Switch2 : Switch  Criteria=u2 > Threshold
  Trigonometric Function : Trigonometry  Operator=tan
  xp [m]1 : InportShadow  Port=2
  yp [m]1 : InportShadow  Port=3
  xc [m] : Outport
  wires:
  yp [m]/1 -> Abs/1
  xp [m]/1 -> Switch/3
  Constant/1 -> Switch/1
  Switch/1 -> Switch1/3
  Abs/1 -> Switch/2
  xp [m]1/1 -> Add/1
  Divide/1 -> Add/2
  yp [m]1/1 -> Divide/1
  Trigonometric Function/1 -> Divide/2
  alfa/1 -> Compare To Constant1/1, Compare To Constant/1, Saturation1/1, Switch2/2, Saturation/1
  Compare To Constant1/1 -> Logical Operator/1
  Compare To Constant/1 -> Logical Operator/2
  Logical Operator/1 -> Switch1/2
  Switch1/1 -> Saturation2/1
  Add/1 -> Switch1/1
  Switch2/1 -> Trigonometric Function/1
  Saturation/1 -> Switch2/1
  Saturation1/1 -> Switch2/3
  Saturation2/1 -> xc [m]/1

== system Experiment_cs/Audi_A8_1/ENABLED/PPS Model/Radar detection/Straight road segment/Relative velocity2 ==
  V [m/s] : Inport
  range [m] : Inport  Port=2
  rangedot [m/s] : Inport  Port=3
  theta [rad] : Inport  Port=4
  theta_p [rad/s] : Inport  Port=5
  Abs{,1..3} (4 alike) : Abs
  Add : Sum  Inputs=++-
  Add2 : Sum  Inputs=-+
  Constant{,1..3} (4 alike) : Constant  Value=0
  Difference : simulink/Discrete/Difference  ICPrevInput=zeros(TISdet,1)  InputProcessing=Inherited  OutMin=[]  OutMax=[]  OutDataType=fixdt(1, 16)  OutScaling=2^-10  DoSatur=off
  Difference1 : simulink/Discrete/Difference  ICPrevInput=zeros(TISdet,1)  InputProcessing=Inherited  OutMin=[]  OutMax=[]  OutDataType=fixdt(1, 16)  OutScaling=2^-10  DoSatur=off
  Difference2 : simulink/Discrete/Difference  ICPrevInput=0.0  InputProcessing=Inherited  OutMin=[]  OutMax=[]  OutDataType=sfix(16)  OutScaling=2^-10  DoSatur=off
  Divide : Product  Inputs=**
  Divide1 : Product  Inputs=***
  Divide4 : Product  Inputs=**
  Divide6 : Product  Inputs=**
  Embedded MATLAB Function1 : MATLAB Function  TreatAsAtomicUnit=on  SystemSampleTime=0.01
  Gain : Gain  Gain=0.01
  Switch : Switch  Threshold=0.5
  Switch1 : Switch  Criteria=u2 > Threshold  Threshold=0.8
  Switch2 : Switch  Threshold=10
  Switch3 : Switch  Criteria=u2 > Threshold  Threshold=10
  Translation : MATLAB Function  TreatAsAtomicUnit=on
  Unit Delay : UnitDelay  InitialCondition=zeros(TISdet,50)  SampleTime=-1
  cos_theta : Trigonometry  Operator=cos
  sin_theta : Trigonometry
  yp' [m/s] : Outport
  xp' [m/s] : Outport  Port=2
  xp [m] : Outport  Port=3
  yp [m] : Outport  Port=4
  Vw [m/s] : Outport  Port=5
  wires:
  rangedot [m/s]/1 -> Divide4/2
  Difference1/1 -> Abs3/1
  Constant3/1 -> Switch3/1
  Constant2/1 -> Switch2/1
  Switch3/1 -> xp' [m/s]/1
  Abs3/1 -> Switch3/2
  Translation/1(xp_dot) -> Difference1/1, Switch3/3
  Abs2/1 -> Switch2/2
  Difference/1 -> Abs2/1
  Switch2/1 -> yp' [m/s]/1
  Switch1/1 -> Switch2/3, Difference/1
  Constant1/1 -> Switch1/3
  Abs1/1 -> Switch1/2
  Gain/1 -> Switch1/1, Abs1/1
  Embedded MATLAB Function1/1(yp2) -> Difference2/1
  Unit Delay/1 -> Embedded MATLAB Function1/3(K1)
  Embedded MATLAB Function1/2(K2) -> Unit Delay/1
  Switch/1 -> Translation/2(xpd)
  Constant/1 -> Switch/3
  Abs/1 -> Switch/2
  Add/1 -> Switch/1, Abs/1
  V [m/s]/1 -> Translation/1(v), Add/1
  Divide1/1 -> Add/3, Add2/2
  Divide4/1 -> Add/2, Add2/1
  Add2/1 -> Vw [m/s]/1
  theta_p [rad/s]/1 -> Divide1/3
  Divide6/1 -> yp [m]/1, Embedded MATLAB Function1/2(yp1)
  cos_theta/1 -> Divide/1, Divide4/1
  sin_theta/1 -> Divide6/2, Divide1/2
  range [m]/1 -> Embedded MATLAB Function1/1(r), Divide1/1, Divide6/1, Divide/2
  Divide/1 -> xp [m]/1
  theta [rad]/1 -> cos_theta/1, sin_theta/1
  Difference2/1 -> Gain/1

== system Experiment_cs/Audi_A8_1/ENABLED/PPS Model/Radar detection/Straight road segment/Saturation1 ==
  TTCin : Inport
  TTCdem_in : Inport  Port=2  SampleTime=1/TISfreq
  Compare To Zero : simulink/Logic and Bit Operations/Compare To Zero  relop=<=  OutDataTypeStr=uint8
  Gain : Gain  Gain=2
  Gain1 : Gain  Gain=ones(TISdet,1)
  Logical Operator : Logic  Operator=OR  AllPortsSameDT=off  OutDataTypeStr=boolean
  Relational Operator : RelationalOperator  Operator=>  OutDataTypeStr=boolean
  Switch : Switch  Criteria=u2 > Threshold  Threshold=0.5
  TTCout : Outport
  TTCdem_out : Outport  Port=2
  wires:
  Gain/1 -> Switch/1, Relational Operator/2
  Gain1/1 -> Gain/1, TTCdem_out/1
  Switch/1 -> TTCout/1
  TTCdem_in/1 -> Gain1/1
  Compare To Zero/1 -> Logical Operator/1
  Relational Operator/1 -> Logical Operator/2
  Logical Operator/1 -> Switch/2
  TTCin/1 -> Switch/3, Compare To Zero/1, Relational Operator/1

== system Experiment_cs/Audi_A8_1/ENABLED/PPS Model/Radar detection/Straight road segment/Saturation2 ==
  TTCin : Inport
  TTCdem_in : Inport  Port=2  SampleTime=1/TISfreq
  Compare To Zero : simulink/Logic and Bit Operations/Compare To Zero  relop=<=  OutDataTypeStr=uint8
  Gain : Gain  Gain=2
  Gain1 : Gain  Gain=ones(TISdet,1)
  Logical Operator : Logic  Operator=OR  AllPortsSameDT=off  OutDataTypeStr=boolean
  Relational Operator : RelationalOperator  Operator=>  OutDataTypeStr=boolean
  Switch : Switch  Criteria=u2 > Threshold  Threshold=0.5
  TTCout : Outport
  TTCdem_out : Outport  Port=2
  wires:
  TTCin/1 -> Relational Operator/1, Compare To Zero/1, Switch/3
  Logical Operator/1 -> Switch/2
  Relational Operator/1 -> Logical Operator/2
  Compare To Zero/1 -> Logical Operator/1
  TTCdem_in/1 -> Gain1/1
  Switch/1 -> TTCout/1
  Gain1/1 -> TTCdem_out/1, Gain/1
  Gain/1 -> Relational Operator/2, Switch/1

== system Experiment_cs/Audi_A8_1/ENABLED/PPS Model/Radar detection/Straight road segment/Saturation3 ==
  TTCin : Inport
  TTCdem_in : Inport  Port=2  SampleTime=1/TISfreq
  Compare To Zero : simulink/Logic and Bit Operations/Compare To Zero  relop=<=  OutDataTypeStr=uint8
  Gain : Gain  Gain=2
  Gain1 : Gain  Gain=ones(TISdet,1)
  Logical Operator : Logic  Operator=OR  AllPortsSameDT=off  OutDataTypeStr=boolean
  Relational Operator : RelationalOperator  Operator=>  OutDataTypeStr=boolean
  Switch : Switch  Criteria=u2 > Threshold  Threshold=0.5
  TTCout : Outport
  TTCdem_out : Outport  Port=2
  wires:
  TTCin/1 -> Relational Operator/1, Compare To Zero/1, Switch/3
  Logical Operator/1 -> Switch/2
  Relational Operator/1 -> Logical Operator/2
  Compare To Zero/1 -> Logical Operator/1
  TTCdem_in/1 -> Gain1/1
  Switch/1 -> TTCout/1
  Gain1/1 -> TTCdem_out/1, Gain/1
  Gain/1 -> Relational Operator/2, Switch/1

== system Experiment_cs/Audi_A8_1/ENABLED/PPS Model/Radar detection/Straight road segment/THETA Derivative1 ==
  range [m] : Inport
  theta [rad] : Inport  Port=2
  Abs1 : Abs
  Deriv correction : MATLAB Function  TreatAsAtomicUnit=on
  Difference1 : simulink/Discrete/Difference  ICPrevInput=0.0  InputProcessing=Inherited  OutMin=[]  OutMax=[]  OutDataType=sfix(16)  OutScaling=2^-10  DoSatur=off
  Difference2 : simulink/Discrete/Difference  ICPrevInput=0.0  InputProcessing=Inherited  OutMin=[]  OutMax=[]  OutDataType=sfix(16)  OutScaling=2^-10  DoSatur=off
  Digital Clock : DigitalClock  SampleTime=1/TISfreq
  Gain : Gain  Gain=0.01
  Gain1 : Gain  Gain=0.01
  Memory : Memory  X0=zeros(TISdet,10,2)  InheritSampleTime=on
  Memory1 : Memory  X0=zeros(TISdet,1)  InheritSampleTime=on
  Memory2 : Memory  X0=zeros(TISdet,1)  InheritSampleTime=on
  Switch : Switch  Threshold=2
  Theta extrapolation : MATLAB Function  TreatAsAtomicUnit=on
  theta_dot [rad/s] : Outport
  wires:
  Memory1/1 -> Deriv correction/2(thp)
  Gain1/1 -> Deriv correction/3(thd)
  Theta extrapolation/1(th2) -> Deriv correction/1(th), Memory1/1, Difference1/1
  range [m]/1 -> Theta extrapolation/1(r)
  Gain/1 -> Theta extrapolation/3(thd)
  Digital Clock/1 -> Theta extrapolation/4(time)
  Memory/1 -> Theta extrapolation/5(K1)
  Theta extrapolation/2(K2) -> Memory/1
  theta [rad]/1 -> Theta extrapolation/2(th1), Difference2/1
  Deriv correction/1(th_dot) -> Switch/3, Abs1/1
  Switch/1 -> Memory2/1, theta_dot [rad/s]/1
  Abs1/1 -> Switch/2
  Memory2/1 -> Switch/1
  Difference2/1 -> Gain/1
  Difference1/1 -> Gain1/1

== system Experiment_cs/Audi_A8_1/ENABLED/PPS Model/Radar detection/Straight road segment/TTC computing1 ==
  xc [m] : Inport
  Vw [m/s] : Inport  Port=2
  Compare To Constant : simulink/Logic and Bit Operations/Compare To Constant  relop===  const=1e-6  OutDataTypeStr=uint8  ZeroCross=off
  Constant : Constant  Value=0
  Data Type Conversion : DataTypeConversion  OutDataTypeStr=double
  Divide : Product  Inputs=/*
  Saturation : Saturate  UpperLimit=inf  LowerLimit=1e-6
  Switch : Switch  Criteria=u2 > Threshold
  Switch1 : Switch  Criteria=u2 > Threshold  Threshold=0.5
  TTC : Outport  InitialOutput=0
  wires:
  Vw [m/s]/1 -> Switch/2, Switch/1
  Constant/1 -> Switch/3, Switch1/1
  Switch/1 -> Saturation/1
  Saturation/1 -> Divide/1, Compare To Constant/1
  Compare To Constant/1 -> Data Type Conversion/1
  xc [m]/1 -> Divide/2
  Divide/1 -> Switch1/3
  Switch1/1 -> TTC/1
  Data Type Conversion/1 -> Switch1/2

== system Experiment_cs/Audi_A8_1/ENABLED/PPS Model/Radar detection/Straight road segment/alfa1 ==
  yp'1 : Inport
  xp' : Inport  Port=2
  Abs : Abs
  Compare To Constant : simulink/Logic and Bit Operations/Compare To Constant  relop===  const=pi/2  OutDataTypeStr=uint8
  Constant : Constant  Value=0
  Switch : Switch  Criteria=u2 > Threshold
  four quadrant atan : Trigonometry  Operator=atan2
  alfa1 : Outport
  wires:
  yp'1/1 -> four quadrant atan/1
  xp'/1 -> four quadrant atan/2
  four quadrant atan/1 -> Abs/1, Switch/3
  Abs/1 -> Compare To Constant/1
  Compare To Constant/1 -> Switch/2
  Constant/1 -> Switch/1
  Switch/1 -> alfa1/1

== system Experiment_cs/Audi_A8_1/ENABLED/Trajectories/Traj2State1/Traj2State2/MuxState ==
  x [m] : Inport
  y [m] : Inport  Port=2
  z [m] : Inport  Port=3
  dx [m/s] : Inport  Port=4
  dy [m/s] : Inport  Port=5
  dz [m/s] : Inport  Port=6
  R [rad] : Inport  Port=7
  P [rad] : Inport  Port=8
  Y [rad] : Inport  Port=9
  Mux : Mux  Inputs=9
  state : Outport
  wires:
  z [m]/1 -> Mux/3
  y [m]/1 -> Mux/2
  x [m]/1 -> Mux/1
  Y [rad]/1 -> Mux/9
  P [rad]/1 -> Mux/8
  R [rad]/1 -> Mux/7
  dz [m/s]/1 -> Mux/6
  dy [m/s]/1 -> Mux/5
  dx [m/s]/1 -> Mux/4
  Mux/1 -> state/1

== system Experiment_cs/Audi_A8_1/ENABLED/Trajectories/Traj2State1/Traj2State2/Traj2MuxState_Ext ==
  Traj : Inport
  Terminator{1..9} (9 alike) : Terminator
  demux : Subsystem
  x [m] : Outport
  y [m] : Outport  Port=2
  z [m] : Outport  Port=3
  dx [m/s] : Outport  Port=4
  dy [m/s] : Outport  Port=5
  dz [m/s] : Outport  Port=6
  R [rad] : Outport  Port=7
  P [rad] : Outport  Port=8
  Y [rad] : Outport  Port=9
  wires:
  demux/9(Y) -> Y [rad]/1
  demux/7(R) -> R [rad]/1
  demux/5(vely) -> dy [m/s]/1
  demux/4(velx) -> dx [m/s]/1
  demux/10(velR) -> Terminator4/1
  demux/11(velP) -> Terminator5/1
  demux/12(velY) -> Terminator1/1
  demux/13(accx) -> Terminator8/1
  demux/14(accy) -> Terminator9/1
  demux/15(accz) -> Terminator7/1
  demux/18(accY) -> Terminator2/1
  demux/16(accR) -> Terminator3/1
  demux/17(accP) -> Terminator6/1
  demux/3(z) -> z [m]/1
  Traj/1 -> demux/1(traj)
  demux/6(velz) -> dz [m/s]/1
  demux/1(x) -> x [m]/1
  demux/2(y) -> y [m]/1
  demux/8(P) -> P [rad]/1

== system Experiment_cs/BMW_Z3_1/ENABLED/Dynamics_Simple/Chassis/Bicycle_model_[XYZ]/Fyi --> Fy / Mz ==
  DeltaWheel_[rad] : Inport
  Fy_f_[N] : Inport  Port=2
  Fy_r_[N] : Inport  Port=3
  Fy : Fcn  Expr=u(2)*cos(u(1)) + u(3)
  Mux1 : Mux  Inputs=3
  Mz : Fcn  Expr=u(2)*p.a*cos(u(1)) - u(3)*p.b
  Fy_[N] : Outport  InitialOutput=0
  Mz_[Nm] : Outport  Port=2  InitialOutput=0
  wires:
  DeltaWheel_[rad]/1 -> Mux1/1  "DeltaWheel_[rad]"
  Mz/1 -> Mz_[Nm]/1
  Fy/1 -> Fy_[N]/1
  Mux1/1 -> Mz/1, Fy/1
  Fy_f_[N]/1 -> Mux1/2
  Fy_r_[N]/1 -> Mux1/3
